simulink model "durumi2_sim_slider_instrument"  (R2022a)
settings: Solver=ode4  StartTime=0.0  StopTime=600  FixedStep=0.01  RelTol=1e-5  EnableMultiTasking=on
InitFcn:
  | durumi2_init
  | x0=zeros(1,12); x0(1)=100; x0(12)=-500;
  | u0=[0;0;0;0.5];
  | 
  | load durumi2_trim_100
undefined symbols (not defined in the file or in its folder): earthRadius, Receive, Send
libraries: simulink_extras x7, aerolibfltsims x3, aerolibanimutils x1
settings Model: Creator=김응태  LastModifiedBy=USer
settings DataIOCC: SaveFormat=Array  SignalLoggingSaveFormat=ModelDataLogs  ReturnWorkspaceOutputs=off  SignalLoggingName=sigsOut
settings OptimizationCC: BooleanDataType=off
settings DebuggingCC: SaveWithParameterizedLinksMsg=none  UnderspecifiedInitializationDetection=Classic  MergeDetectMultiDrivingBlocksExec=none  SignalResolutionControl=TryResolveAllWithWarning  MultiTaskDSMMsg=warning  MultiTaskCondExecSysMsg=none  UnconnectedInputMsg=warning  UnconnectedOutputMsg=warning  UnconnectedLineMsg=warning
settings HardwareCC: ProdBitPerPointer=32  ProdBitPerSizeT=32  ProdBitPerPtrDiffT=32  ProdLargestAtomicFloat=None  ProdIntDivRoundTo=Undefined  ProdEndianess=Unspecified  ProdWordSize=32  ProdHWDeviceType=32-bit Generic  TargetUnknown=on
settings ModelReferenceCC: PropagateSignalLabelsOutOfModel=off
settings GRTTargetCC: CombineOutputUpdateFcns=off  GRTInterface=on
settings ConfigComp: CovMetricSettings=dw  CovSaveCumulativeToWorkspaceVar=on  CovSaveSingleToWorkspaceVar=on

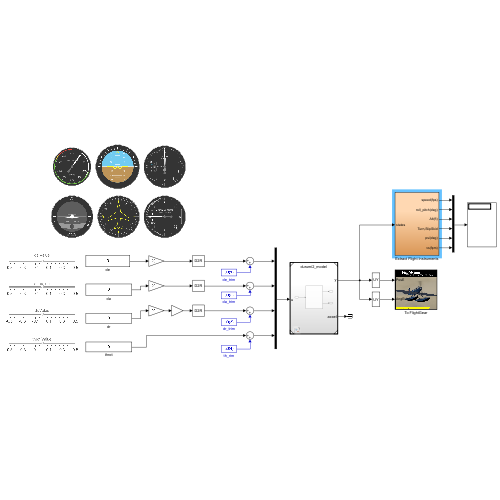
[thumbnail: Simulink's stored preview of the top-level diagram]
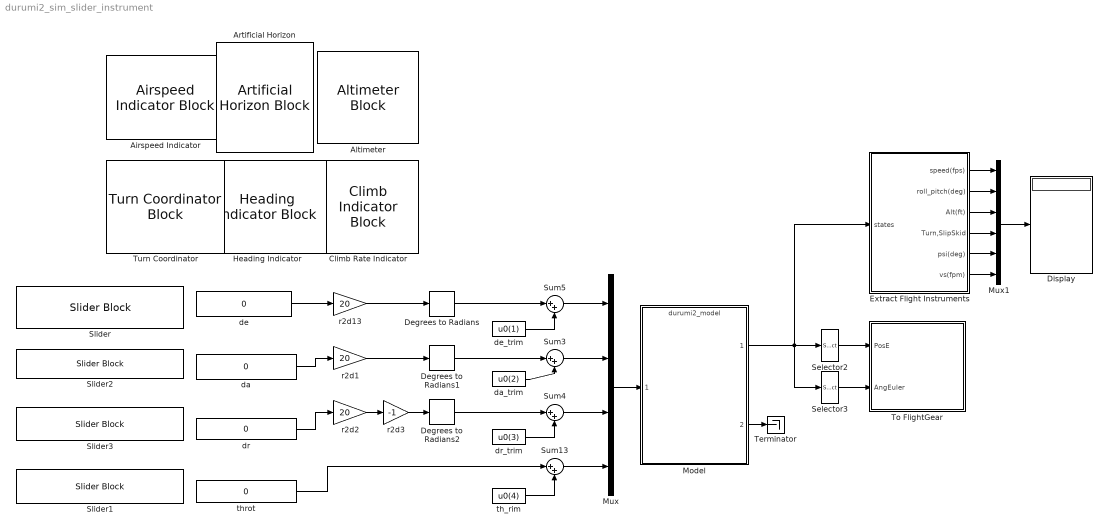
== system durumi2_sim_slider_instrument ==
  Airspeed Indicator : AirspeedIndicatorBlock  LabelPosition=Hide  ScaleMin=0  ScaleMax=450
  Altimeter : AltimeterBlock  LabelPosition=Hide
  Artificial Horizon : ArtificialHorizonBlock  LabelPosition=Hide
  Climb Rate Indicator : ClimbIndicatorBlock  LabelPosition=Hide  ScaleMax=16000
  Degrees to Radians : simulink_extras/Transformations/Degrees to Radians
  Degrees to Radians1 : simulink_extras/Transformations/Degrees to Radians
  Degrees to Radians2 : simulink_extras/Transformations/Degrees to Radians
  Display : Display
  Extract Flight Instruments : Subsystem
  Heading Indicator : HeadingIndicatorBlock  LabelPosition=Hide
  Model : ModelReference  ModelNameDialog=durumi2_model.slx  SimulationMode=Normal  ModelReferenceVersion=1.75
  Mux : Mux
  Mux1 : Mux  Inputs=6
  Selector2 : Selector  InputPortWidth=12  IndexOptions=Index vector (dialog)  Indices=10:12  OutputSizes=1
  Selector3 : Selector  InputPortWidth=12  IndexOptions=Index vector (dialog)  Indices=7:9  OutputSizes=1
  Slider{,1..3} (4 alike) : SliderBlock  ScaleMin=-0.5  ScaleMax=0.5
  Sum{3..5,13} (4 alike) : Sum  Inputs=|++  InputSameDT=on  OutDataTypeStr=Inherit: Same as first input
  Terminator : Terminator
  To FlightGear : Subsystem
      mask Display: image('FlightGear.png'); % Use "Edit Image" on toolstrip to change.
  Turn Coordinator : TurnCoordinatorBlock  LabelPosition=Hide
  da : Constant  Value=0
  da_trim : Constant  Value=u0(2)  VectorParams1D=off
  de : Constant  Value=0
  de_trim : Constant  Value=u0(1)  VectorParams1D=off
  dr : Constant  Value=0
  dr_trim : Constant  Value=u0(3)  VectorParams1D=off
  r2d1 : Gain  Gain=20  OutDataTypeStr=Inherit: Same as input  ParamDataTypeStr=Inherit: Same as input
  r2d13 : Gain  Gain=20  OutDataTypeStr=Inherit: Same as input  ParamDataTypeStr=Inherit: Same as input
  r2d2 : Gain  Gain=20  OutDataTypeStr=Inherit: Same as input  ParamDataTypeStr=Inherit: Same as input
  r2d3 : Gain  Gain=-1  OutDataTypeStr=Inherit: Same as input  ParamDataTypeStr=Inherit: Same as input
  th_rim : Constant  Value=u0(4)  VectorParams1D=off
  throt : Constant  Value=0
  wires:
  Sum4/1 -> Mux/3
  dr_trim/1 -> Sum4/2
  Sum3/1 -> Mux/2
  Mux/1 -> Model/1
  Sum13/1 -> Mux/4
  de_trim/1 -> Sum5/2
  th_rim/1 -> Sum13/2
  dr/1 -> r2d2/1
  Sum5/1 -> Mux/1
  r2d1/1 -> Degrees to Radians1/1
  da_trim/1 -> Sum3/2
  da/1 -> r2d1/1
  de/1 -> r2d13/1
  Selector3/1 -> To FlightGear/2(AngEuler)
  Selector2/1 -> To FlightGear/1(PosE)
  Degrees to Radians/1 -> Sum5/1
  Degrees to Radians1/1 -> Sum3/1
  Degrees to Radians2/1 -> Sum4/1
  throt/1 -> Sum13/1
  r2d2/1 -> r2d3/1
  r2d13/1 -> Degrees to Radians/1
  Model/2 -> Terminator/1
  Extract Flight Instruments/3(Alt(ft)) -> Mux1/3
  Extract Flight Instruments/1(speed(fps)) -> Mux1/1
  Extract Flight Instruments/2(roll_pitch(deg)) -> Mux1/2
  Extract Flight Instruments/6(vs(fpm)) -> Mux1/6
  Extract Flight Instruments/4(Turn,SlipSkid) -> Mux1/4
  Model/1 -> Extract Flight Instruments/1(states), Selector3/1, Selector2/1
  Extract Flight Instruments/5(psi(deg)) -> Mux1/5
  Mux1/1 -> Display/1
  r2d3/1 -> Degrees to Radians2/1

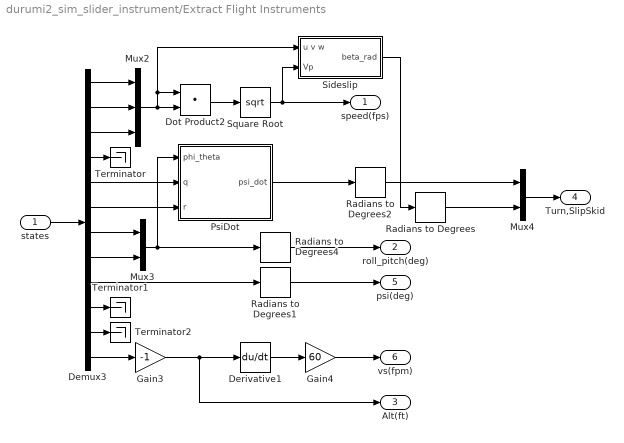
== system durumi2_sim_slider_instrument/Extract Flight Instruments ==
  states : Inport
  Demux3 : Demux  Outputs=12
  Derivative1 : Derivative
  Dot Product2 : DotProduct  OutDataTypeStr=Inherit: Inherit via internal rule
  Gain3 : Gain  Gain=-1
  Gain4 : Gain  Gain=60
  Mux2 : Mux  Inputs=3
  Mux3 : Mux  Inputs=2
  Mux4 : Mux  Inputs=2
  PsiDot : Subsystem
  Radians to Degrees{,1..2,4} (4 alike) : simulink_extras/Transformations/Radians to Degrees
  Sideslip : Subsystem
  Square Root : Sqrt
  Terminator : Terminator
  Terminator1 : Terminator
  Terminator2 : Terminator
  speed(fps) : Outport
  roll_pitch(deg) : Outport  Port=2
  Alt(ft) : Outport  Port=3
  Turn,SlipSkid : Outport  Port=4
  psi(deg) : Outport  Port=5
  vs(fpm) : Outport  Port=6
  wires:
  Radians to Degrees1/1 -> psi(deg)/1
  Derivative1/1 -> Gain4/1
  Mux2/1 -> Sideslip/1(u v w), Dot Product2/1, Dot Product2/2
  Radians to Degrees4/1 -> roll_pitch(deg)/1
  Mux3/1 -> Radians to Degrees4/1, PsiDot/1(phi_theta)
  Gain4/1 -> vs(fpm)/1
  Dot Product2/1 -> Square Root/1
  Gain3/1 -> Derivative1/1, Alt(ft)/1
  Demux3/12 -> Gain3/1
  Demux3/9 -> Radians to Degrees1/1
  Square Root/1 -> speed(fps)/1, Sideslip/2(Vp)
  states/1 -> Demux3/1
  Demux3/1 -> Mux2/1
  Demux3/2 -> Mux2/2
  Demux3/3 -> Mux2/3
  Demux3/7 -> Mux3/1
  Demux3/8 -> Mux3/2
  Demux3/5 -> PsiDot/2(q)
  Demux3/6 -> PsiDot/3(r)
  PsiDot/1(psi_dot) -> Radians to Degrees2/1
  Mux4/1 -> Turn,SlipSkid/1
  Demux3/4 -> Terminator/1
  Demux3/10 -> Terminator1/1
  Demux3/11 -> Terminator2/1
  Radians to Degrees2/1 -> Mux4/1
  Radians to Degrees/1 -> Mux4/2
  Sideslip/1(beta_rad) -> Radians to Degrees/1

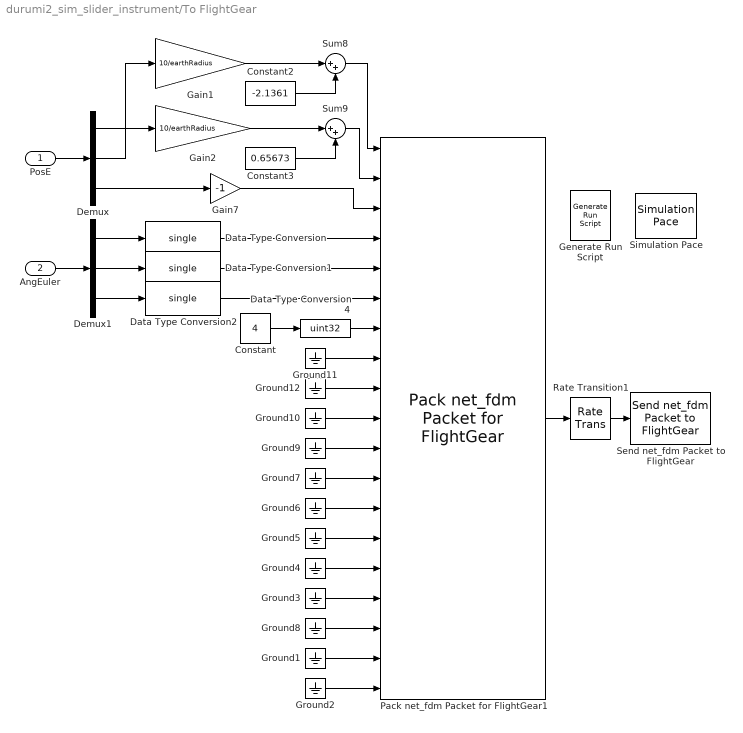
== system durumi2_sim_slider_instrument/To FlightGear ==
  PosE : Inport
  AngEuler : Inport  Port=2
  Constant : Constant  Value=4
  Constant2 : Constant  Value=-2.1361  VectorParams1D=off
  Constant3 : Constant  Value=0.65673  VectorParams1D=off
  Data Type Conversion : DataTypeConversion  OutDataTypeStr=single  RndMeth=Floor
  Data Type Conversion1 : DataTypeConversion  OutDataTypeStr=single  RndMeth=Floor
  Data Type Conversion2 : DataTypeConversion  OutDataTypeStr=single  RndMeth=Floor
  Data Type Conversion4 : DataTypeConversion  OutDataTypeStr=uint32  SaturateOnIntegerOverflow=off  RndMeth=Floor
  Demux : Demux  Outputs=3
  Demux1 : Demux  Outputs=3
  Gain1 : Gain  Gain=10/earthRadius
  Gain2 : Gain  Gain=10/earthRadius
  Gain7 : Gain  Gain=-1
  Generate Run Script : aerolibfltsims/Generate Run Script  Architecture=Default  dataFlow=Send-Receive  GeometryModelName=Rotor4  AirportId=KSF0  RunwayId=10L  InitialAltitude=0  InitialHeading=0  OffsetDistance=0  OffsetAzimuth=0  InstallScenery=off  DisableShaders=off  OriginAddress=127.0.0.1  DestinationPort=5502  OriginPort=5505  LocalAddress=127.0.0.1  OutputFileName=runfg.bat  FlightGearBaseDirectory=C:\Program Files\FlightGear 2016.1.2
  Ground{1..12} (12 alike) : Ground
  Pack net_fdm Packet for FlightGear1 : aerolibfltsims/Pack net_fdm Packet for FlightGear  FlightGearVersion=v2016.1  ShowPositionAttitudeInputs=on  ShowVelocityAccelerationInputs=off  ShowControlSurfacePositionInputs=off  ShowEngineFuelInputs=on  ShowLandingGearInputs=off  ShowEnvironmentInputs=off  SampleTime=0.01  packetVersion=24
      settings: SourceProductBaseCode=AE
  Rate Transition1 : RateTransition
  Send net_fdm Packet to FlightGear : aerolibfltsims/Send net_fdm Packet to FlightGear  DestinationIpAddress=127.0.0.1  DestinationPort=5502  LocalIpPort=-1  varLen=off  SampleTime=0.01
      settings: SourceProductBaseCode=AE
  Simulation Pace : aerolibanimutils/Simulation Pace  SimulationPace=1  SleepMode=MATLAB Thread  OutputPaceError=off  SampleTime=-1
      settings: AttributesFormatString=%<SimulationPace> sec/sec
  Sum8 : Sum  Inputs=|++
  Sum9 : Sum  Inputs=|++
  wires:
  AngEuler/1 -> Demux1/1
  PosE/1 -> Demux/1
  Demux1/1 -> Data Type Conversion/1
  Demux/1 -> Gain2/1
  Constant/1 -> Data Type Conversion4/1
  Demux/3 -> Gain7/1
  Sum9/1 -> Pack net_fdm Packet for FlightGear1/2
  Sum8/1 -> Pack net_fdm Packet for FlightGear1/1
  Data Type Conversion/1 -> Pack net_fdm Packet for FlightGear1/4
  Data Type Conversion1/1 -> Pack net_fdm Packet for FlightGear1/5
  Data Type Conversion2/1 -> Pack net_fdm Packet for FlightGear1/6
  Data Type Conversion4/1 -> Pack net_fdm Packet for FlightGear1/7
  Demux1/2 -> Data Type Conversion1/1
  Pack net_fdm Packet for FlightGear1/1 -> Rate Transition1/1
  Gain2/1 -> Sum9/1
  Gain1/1 -> Sum8/1
  Demux1/3 -> Data Type Conversion2/1
  Demux/2 -> Gain1/1
  Rate Transition1/1 -> Send net_fdm Packet to FlightGear/1
  Constant2/1 -> Sum8/2
  Constant3/1 -> Sum9/2
  Gain7/1 -> Pack net_fdm Packet for FlightGear1/3
  Ground8/1 -> Pack net_fdm Packet for FlightGear1/17
  Ground1/1 -> Pack net_fdm Packet for FlightGear1/18
  Ground2/1 -> Pack net_fdm Packet for FlightGear1/19
  Ground11/1 -> Pack net_fdm Packet for FlightGear1/8
  Ground10/1 -> Pack net_fdm Packet for FlightGear1/10
  Ground9/1 -> Pack net_fdm Packet for FlightGear1/11
  Ground7/1 -> Pack net_fdm Packet for FlightGear1/12
  Ground6/1 -> Pack net_fdm Packet for FlightGear1/13
  Ground5/1 -> Pack net_fdm Packet for FlightGear1/14
  Ground4/1 -> Pack net_fdm Packet for FlightGear1/15
  Ground3/1 -> Pack net_fdm Packet for FlightGear1/16
  Ground12/1 -> Pack net_fdm Packet for FlightGear1/9

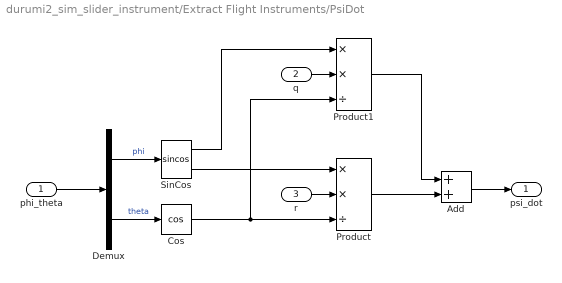
== system durumi2_sim_slider_instrument/Extract Flight Instruments/PsiDot ==
  phi_theta : Inport
  q : Inport  Port=2
  r : Inport  Port=3
  Add : Sum
  Cos : Trigonometry  Operator=cos
  Demux : Demux  Outputs=2
  Product : Product  Inputs=**/
  Product1 : Product  Inputs=**/
  SinCos : Trigonometry  Operator=sincos
  psi_dot : Outport
  wires:
  Demux/1 -> SinCos/1  "phi"
  Demux/2 -> Cos/1  "theta"
  Add/1 -> psi_dot/1
  Cos/1 -> Product/3, Product1/3
  q/1 -> Product1/2
  r/1 -> Product/2
  Product1/1 -> Add/1
  Product/1 -> Add/2
  SinCos/1 -> Product1/1
  SinCos/2 -> Product/1
  phi_theta/1 -> Demux/1

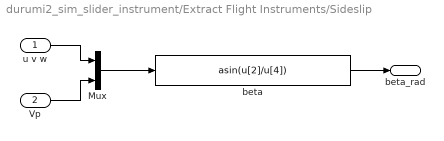
== system durumi2_sim_slider_instrument/Extract Flight Instruments/Sideslip ==
  u v w : Inport
  Vp : Inport  Port=2
  Mux : Mux  Inputs=2
  beta : Fcn  Expr=asin(u[2]/u[4])
  beta_rad : Outport  InitialOutput=0  VectorParamsAs1DForOutWhenUnconnected=off
  wires:
  Mux/1 -> beta/1
  beta/1 -> beta_rad/1
  Vp/1 -> Mux/2
  u v w/1 -> Mux/1
